simulink model "fcs_archi"  (R2023b)
settings: Solver=FixedStepAuto  StartTime=0.0  StopTime=10.0  FixedStep=5e-5  RelTol=1e-3
values from neighbouring files (symbols this model uses):
  density_of_air = 1.2    [fcs_spec.sldd]
  f_Baro_Alt = 50.0    [fcs_spec.sldd]
  f_GPS = 10.0    [fcs_spec.sldd]
  f_IMU = 1000.0    [fcs_spec.sldd]
  f_Mag = 50.0    [fcs_spec.sldd]
  f_Pitot = 50.0    [fcs_spec.sldd]
  g = 9.8    [fcs_spec.sldd]
undefined symbols (not defined in the file or in its folder): Climb_Alt, DiscIntNeverNeededParam, f_fidr, f_inner_loop, f_outer_loop, f_sensor_acquisition, Pitch_Angle_Max, Pitch_Angle_Min, Pitch_Rate_Max, Roll_Angle_Max, Roll_Rate_Max, Sensor_Mode, Takeoff_Alt, Takeoff_Spd, Yaw_Rate_Max
libraries: dspfdesign x5, simulink x3, sharedtransform x1
(part 2 of 2)

== system fcs_archi/FCS/Sensor_Acquisition_Task/Data_Acquisition/Signal_Validaton/Subsystem4 ==
  Max : Inport
  Signal : Inport  Port=2
  Min : Inport  Port=3
  AND : Logic  Inputs=3  IconShape=distinctive  AllPortsSameDT=off  OutDataTypeStr=boolean
  AND1 : Logic  Inputs=1  IconShape=distinctive  AllPortsSameDT=off  OutDataTypeStr=boolean
  Relational Operator : RelationalOperator  Operator=<=  OutDataTypeStr=boolean  RndMeth=Simplest  InputSameDT=off
  Relational Operator1 : RelationalOperator  OutDataTypeStr=boolean  RndMeth=Simplest  InputSameDT=off
  Relational Operator2 : RelationalOperator  Operator=isFinite  OutDataTypeStr=boolean  RndMeth=Simplest  InputSameDT=off
  Validity : Outport
  wires:
  AND/1 -> AND1/1
  Relational Operator1/1 -> AND/2
  Signal/1 -> Relational Operator/1, Relational Operator2/1, Relational Operator1/1
  Relational Operator2/1 -> AND/3
  Relational Operator/1 -> AND/1
  Max/1 -> Relational Operator/2
  Min/1 -> Relational Operator1/2
  AND1/1 -> Validity/1

== matlab function fcs_archi/FCS/FDIR_Task/Sensor_FDIR/Notify_D2_Sensor_State/notify_D2 ==
  data: sensor_state input
function notify_d2_sensor_state(sensor_state)

    for i = 1:3:length(sensor_state)
        if sensor_state(i) == true
            if i == 1
                disp('All IMU degraded')
            elseif i == 4
                disp('All Mag degraded')
            elseif i == 7
                disp('All GPS degraded')
            elseif i == 10
                disp('All Baro_Alt degraded')
            else
                disp('All Pitot degraded')
            end
        end
    end

== matlab function fcs_archi/FCS/FDIR_Task/Sensor_FDIR/Notify_D1_Sensor_State/notify_D1 ==
  data: sensor_state input
function notify_sensor_state(sensor_state)

    for i = 1:length(sensor_state)
        if sensor_state(i) == true
            if i >= 1 && i <= 3
                disp('IMU_%d degraded', i)
            elseif i >= 4 && i <= 6
                disp('Mag_%d degraded', i)
            elseif i >= 7 && i <= 9
                disp('GPS_%d degraded', i)
            elseif i >= 10 && i <= 12
                disp('Baro_Alt_%d degraded', i)
            else
                disp('Pitot_%d degraded', i)
            end
        end
    end

== stateflow chart fcs_archi/FCS/FDIR_Task/Sensor_FDIR/Measurement_Health ==
  state Sensor_Mode
    state Critical
      en: Sensor_Mode = Critical
    state Stabilize
      en: Sensor_Mode =  Stabilize
    state Healthy_Mode
      state No_GPS
        en: Sensor_Mode = No_GPS
      state Compensated_Mode
        du: Is_GPS_compensation_needed = (Baro_Alt_Mode == D2 || Mag_Mode == D2 || Pitot_Mode == D2)
        state GPS_Alt
          en: Sensor_Mode = GPS_Alt
        state GPS_Hdg
          en: Sensor_Mode = GPS_Hdg
        state GPS_Spd
          en: Sensor_Mode = GPS_Spd
        state GPS_Alt_Spd
          en: Sensor_Mode = GPS_Alt_Spd
        state GPS_Spd_Hdg
          en: Sensor_Mode = GPS_Spd_Hdg
        state GPS_Alt_Hdg
          en: Sensor_Mode = GPS_Alt_Hdg
        state GPS_Compensated
          en: Sensor_Mode = GPS_Compensated
        (junction 155) -> GPS_Alt [order 1] : [Baro_Alt_Mode == D2 && Pitot_Mode ~= D2 && Mag_Mode ~= D2]
        (junction 155) -> GPS_Hdg [order 7] : [Baro_Alt_Mode ~= D2 && Pitot_Mode ~= D2 && Mag_Mode == D2]
        (junction 155) -> GPS_Spd [order 6] : [Baro_Alt_Mode ~= D2 && Pitot_Mode == D2 && Mag_Mode ~= D2]
        (junction 155) -> GPS_Compensated [order 2] : [Baro_Alt_Mode == D2 && Pitot_Mode == D2 && Mag_Mode == D2]
        (junction 155) -> GPS_Spd_Hdg [order 4] : [Baro_Alt_Mode ~= D2 && Pitot_Mode == D2 && Mag_Mode == D2]
        (junction 155) -> GPS_Alt_Hdg [order 3] : [Baro_Alt_Mode == D2 && Pitot_Mode ~= D2 && Mag_Mode == D2]
        (junction 155) -> GPS_Alt_Spd [order 5] : [Baro_Alt_Mode == D2 && Pitot_Mode == D2 && Mag_Mode ~= D2]
      state Healthy
        en: Sensor_Mode = Healthy
        du: Is_GPS_compensation_needed = (Baro_Alt_Mode == D2 || Mag_Mode == D2 || Pitot_Mode == D2)
      (junction 88) -> (junction 91) [order 2] : [GPS_Mode == D2]
      (junction 91) -> No_GPS
      Healthy -> (junction 91) [order 1] : [GPS_Mode == D2]
      (junction 88) -> (junction 42) [order 1] : [GPS_Mode ~= D2]
      Compensated_Mode -> (junction 91) [order 2] : [GPS_Mode == D2]
      No_GPS -> (junction 42) : [GPS_Mode ~= D2]
      (junction 42) -> (junction 94) [order 1] : [Is_GPS_compensation_needed]
      (junction 42) -> Healthy [order 2] : [~Is_GPS_compensation_needed]
      (junction 94) -> (junction 155)
      Healthy -> (junction 94) [order 2] : [Is_GPS_compensation_needed]
      (default) -> Healthy
      Compensated_Mode -> Healthy [order 1] : [~Is_GPS_compensation_needed]
    (default) -> Critical
    Stabilize -> Critical [order 2] : [GPS_Mode == D2]
    Critical -> Stabilize [order 2] : [GPS_Mode ~= D2]
    Stabilize -> (junction 120) [order 1] : [IMU_Mode ~= D2]
    (junction 38) -> Stabilize [order 1] : [GPS_Mode ~= D2]
    Critical -> (junction 120) [order 1] : [IMU_Mode ~= D2]
    (junction 38) -> Critical [order 2] : [GPS_Mode == D2]
    Healthy_Mode -> (junction 38) : [IMU_Mode == D2]
    (junction 120) -> (junction 88)
  data: IMU_Mode input Enum: Sensor_Mode; Baro_Alt_Mode input Enum: Sensor_Mode; Mag_Mode input Enum: Sensor_Mode; Pitot_Mode input Enum: Sensor_Mode; GPS_Mode input Enum: Sensor_Mode; Sensor_Mode output Enum: Sensor_FDIR_Mode; Critical local Enum: Sensor_FDIR_Mode =Sensor_FDIR_Mode('Critical'); Stabilize local Enum: Sensor_FDIR_Mode =Sensor_FDIR_Mode('Stabilize'); D2 local Enum: Sensor_Mode =Sensor_Mode('D2'); Is_GPS_compensation_needed local boolean =false

== stateflow chart fcs_archi/FCS/FDIR_Task/Sensor_FDIR/Notify_D1 ==
  state No_D1
    en: Notify_D1 = false
  state D1
    en: Notify_D1 = true
  No_D1 -> D1 : [IMU_Mode == D1 || GPS_Mode == D1 || Mag_Mode == D1 || Baro_Alt_Mode == D1 || Pitot_Mode == D1 ]
  (default) -> No_D1
  D1 -> No_D1 : [~(IMU_Mode == D1 || GPS_Mode == D1 || Mag_Mode == D1 || Baro_Alt_Mode == D1 || Pitot_Mode == D1 )]
  data: IMU_Mode input Enum: Sensor_Mode; Baro_Alt_Mode input Enum: Sensor_Mode; Mag_Mode input Enum: Sensor_Mode; Pitot_Mode input Enum: Sensor_Mode; GPS_Mode input Enum: Sensor_Mode; Notify_D1 output boolean

== matlab function fcs_archi/FCS/Kin_State_Propagation/UAV kinematics/MATLAB Function ==
  data: w input; roll input; euler_angle_rate output; pitch input
function euler_angle_rate = convert_angular_vel2euler_rate(w, roll, pitch)
p = w(1);
q = w(2);
r = w(3);

euler_angle_rate = [p + (q*sin(roll)+r*cos(roll))*tan(pitch),
                    q*cos(roll)-r*sin(roll),
                    (q*sin(roll)+r*cos(roll)/cos(pitch))];

== matlab function fcs_archi/FCS/FDIR_Task/Actuator_FDIR ==
  data: elevator_sat input; aileron_sat input; rudder_sat input; esc_sat input
function Notify_Actuator_Saturation(elevator_sat,aileron_sat, rudder_sat, esc_sat)
    if elevator_sat
        disp('Elevator Servo saturated')
    end

    if aileron_sat
        disp('Aileron Servo saturated')
    end

    if rudder_sat
        disp('Rudder Servo saturated')
    end

    if esc_sat
        disp('ESC saturated')
    end

end

== stateflow chart fcs_archi/FCS/Mission_Manager_Task/Flight_Phase_Manager ==
  state PREFLIGHT
    en: Flight_Phase = PREFLIGHT
  state TAKEOFF
    en: Flight_Phase =TAKEOFF
  state CLIMB
    en: Flight_Phase = CLIMB
  state LANDING
    en: Flight_Phase = LANDING
  state CRUISE
    en: Flight_Phase = CRUISE
  note: [Alt <= Target_Alt && Alt <= Landing_Alt]
  state DESCENT
    en: Flight_Phase = DESCENT
  (default) -> PREFLIGHT
  PREFLIGHT -> TAKEOFF : [Spd > Takeoff_Spd && Alt > Takeoff_Alt]
  LANDING -> PREFLIGHT : [Alt <= 0.01 && Spd <= 0.01]
  TAKEOFF -> CLIMB : [Alt > Climb_Alt]
  CRUISE -> CLIMB [order 1] : [Alt < (Target_Alt - 10)]
  CLIMB -> CRUISE : [Alt >= (Target_Alt - 10) && Alt <= (Target_Alt + 10)]
  DESCENT -> LANDING [order 2]
  CRUISE -> DESCENT [order 2] : [Alt > (Target_Alt + 10)]
  DESCENT -> CRUISE [order 1] : [Alt >= (Target_Alt - 10) && Alt <= (Target_Alt + 10)]
  data: Flight_Phase output Enum: Flight_Phase; Spd input; Alt input; Takeoff_Alt parameter double; Takeoff_Spd parameter; Target_Alt input; Climb_Alt parameter
